simulink model "part2a"  (R2013a)
settings: Solver=ode45  StartTime=0.0  StopTime=t_end  RelTol=1e-5
values from neighbouring files (symbols this model uses):
  c = Beq + Bemf    (= 10.2235639816)    [lab1.m]
  gamma = (nu_g*Kg*nu_m*Kt)/(Rm*rmp)    (= 1.72354330709)    [lab1.m]
  k = 10    [lab1.m]
  m = M + Mj    (= 1.07312664145)    [lab1.m]
  r0 = 0.4    [lab1.m]
settings Model: Creator=Willdog  LastModifiedBy=Willdog

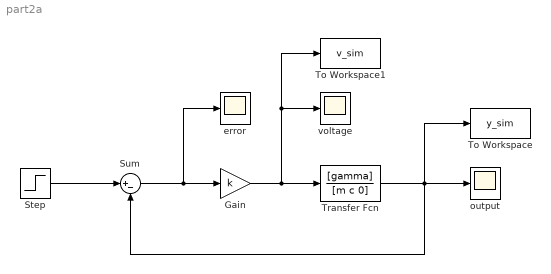
== system part2a ==
  Gain : Gain  Gain=k
  Step : Step  Time=0  After=r0  SampleTime=0
  Sum : Sum  Inputs=|+-
  To Workspace : ToWorkspace  VariableName=y_sim  SampleTime=-1  SaveFormat=Timeseries
  To Workspace1 : ToWorkspace  VariableName=v_sim  SampleTime=-1  SaveFormat=Timeseries
  Transfer Fcn : TransferFcn  Numerator=[gamma]  Denominator=[m c 0]
  error : Scope
  output : Scope
  voltage : Scope
      settings: SaveName=ScopeData2
  wires:
  Step/1 -> Sum/1
  Sum/1 -> error/1, Gain/1
  Gain/1 -> To Workspace1/1, voltage/1, Transfer Fcn/1
  Transfer Fcn/1 -> Sum/2, To Workspace/1, output/1
